simulink model "P4Model"  (R2023b)
settings: Solver=FixedStepAuto  StartTime=0.0  StopTime=3600  FixedStep=0.1  RelTol=1e-3
values from neighbouring files (symbols this model uses):
  psi = [0]    [Project2Init.m]
  x = [0]    [Project2Init.m]
  y = [0]    [Project2Init.m]
undefined symbols (not defined in the file or in its folder): batData, carData, motorData, rps2rpm
libraries: slpidlib x1
settings Model: Creator=ronal  LastModifiedBy=ronal
settings DebuggingCC: AlgebraicLoopMsg=none

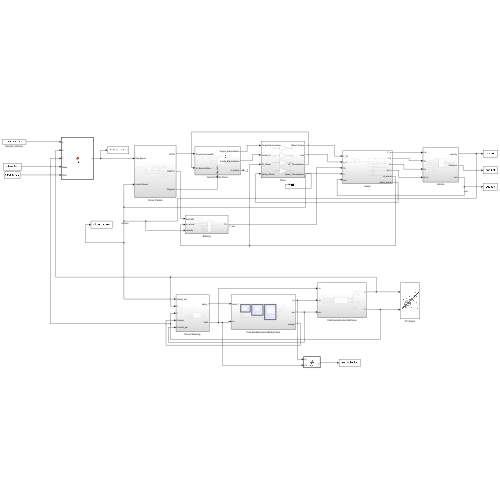
[thumbnail: Simulink's stored preview of the top-level diagram]
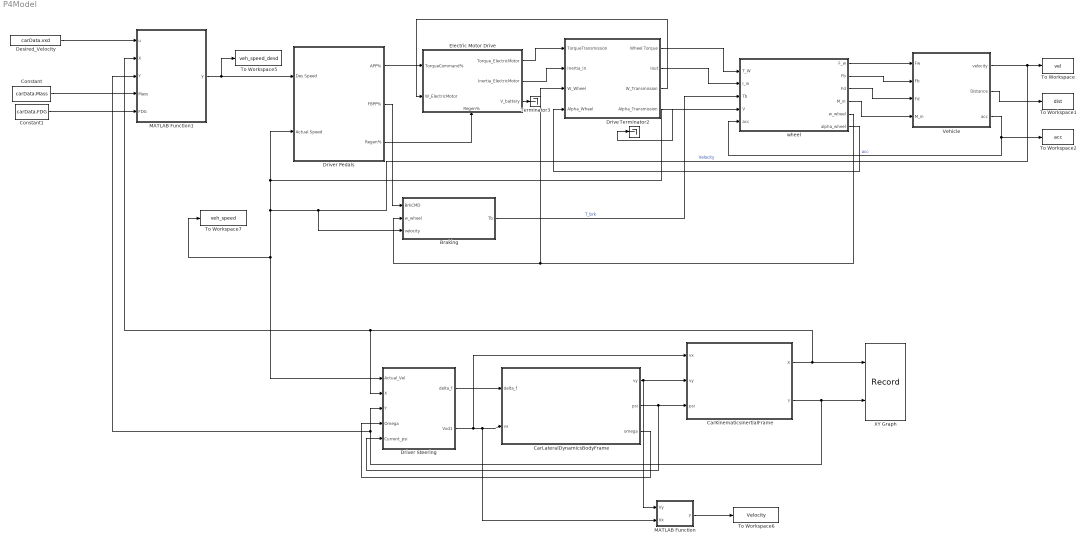
== system P4Model ==
  Braking : Subsystem
  CarKinematicsInertialFrame : Subsystem
  CarLateralDynamicsBodyFrame : Subsystem
  Constant : Constant  Value=carData.Mass
  Constant1 : Constant  Value=carData.FDG
  Desired_Velocity : Constant  Value=carData.vxd
  Drive : Subsystem
  "Driver Pedals " : Subsystem
  Driver Steering : Subsystem
  Electric Motor Drive : Subsystem
      settings: PortSchema="{\"entries\":[{\"content\":{\"sides\":[{\"content\":{\"connectorIds\":[\"In1\",\"In2\"]},\"type\":\"ConnectorPlacement.EquallySpacedRectSide\",\"uuid\":\"06f5b496-3bf6-4a8b-aebb-c7eaab5f1ccf\"},{\"content\":{\"connectorIds\":[\"Out1\",\"Out2\",\"Out3\"],\"side\":\"RIGHT\"},\"type\":\"ConnectorPlacement.EquallySpacedRectSide\",\"uuid\":\"1c240108-0efa-470d-9e35-d17d0925c84e\"},{\"content\":{\"side\":\"TOP\"},\"type\":\"ConnectorPlacement.EquallySpacedRectSide\",\"uuid\":\"0076995f-d270-4ea1-a86d-c1644fbb58c6\"},{\"content\":{\"connectorIds\":[\"In3\"],\"side\":\"BOTTOM\"},\"type\":\"ConnectorPlacement.EquallySpacedRectSide\",\"uuid\":\"f7a02404-3e3b-4c45-bbfb-e79306aab2e1\"}]},\"type\":\"ConnectorPlacement.EquallySpacedConnector\",\"uuid\":\"8c37f1ab-19c5-40e9-996c-a411e99a53bc\"}],\"packageUris\":[\"http://schema.mathworks.com/mf0/Connector/R2020b\"],\"version\":\"1.0\"}"
  MATLAB Function : MATLAB Function  TreatAsAtomicUnit=on
  MATLAB Function1 : MATLAB Function  TreatAsAtomicUnit=on
  Terminator2 : Terminator
  Terminator3 : Terminator
  To Workspace : ToWorkspace  VariableName=vel  SaveFormat=Timeseries  SampleTime=-1
  To Workspace1 : ToWorkspace  VariableName=dist  SaveFormat=Timeseries  SampleTime=-1
  To Workspace2 : ToWorkspace  VariableName=acc  SaveFormat=Timeseries  SampleTime=-1
  To Workspace5 : ToWorkspace  VariableName=veh_speed_desd  SaveFormat=Timeseries  SampleTime=-1
  To Workspace6 : ToWorkspace  VariableName=Velocity  SaveFormat=Timeseries  SampleTime=-1
  To Workspace7 : ToWorkspace  VariableName=veh_speed  SaveFormat=Timeseries  SampleTime=-1
  Vehicle : Subsystem
  XY Graph : Record  FileSettingsInternal="{\"entries\":[{\"content\":{\"excelSettings\":{\"content\":{},\"type\":\"Streamout.ExcelSettings\"}},\"type\":\"Streamout.FileSettingStorage\",\"uuid\":\"\"}],\"packageUris\":[\"http:\\/\\/schema.mathworks.com\\/mf0\\/streamout_blocks\\/R2020a\"],\"version\":\"1.0\"}"  Layout=[1 1]  SignalsInternal="{\"entries\":[{\"content\":{\"signals\":[{\"content\":{\"blockPath\":[],\"dimensions\":[1],\"domain\":\"\",\"lineColor\":\"#0072bd\",\"plots\":[1],\"port\":1,\"sid\":[\"\"],\"signalID\":2554,\"signalName\":\"CarKinematicsInertialFrame:1\"},\"type\":\"RecordBlkView.Signal\",\"uuid\":\"\"},{\"content\":{\"blockPath\":[],\"dimensions\":[1],\"domain\":\"\",\"lineColor\":\"#ff13a6\",\"plots\":[1],\"port\":2,\"sid\":[\"\"],\"signalID\":2558,\"signalName\":\"CarKinematicsInertialFrame:2\"},\"type\":\"RecordBlkView.Signal\",\"uuid\":\"\"}]},\"type\":\"RecordBlkView.InputSignals\",\"uuid\":\"\"}],\"packageUris\":[\"http:\\/\\/schema.mathworks.com\\/mf0\\/streamout_blocks\\/R2020a\"],\"version\":\"1.0\"}"  VisualizationBindings="{\"xyplotplugin\":{\"info\":[{\"series\":[{\"bindingParametersList\":[{\"parameter\":\"Y-Axis\",\"signalID\":2558,\"signalName\":\"CarKinematicsInertialFrame:2\"},{\"parameter\":\"X-Axis\",\"signalID\":2554,\"signalName\":\"CarKinematicsInertialFrame:1\"}],\"seriesID\":48790}],\"subplotID\":1}]}}"  CompatibilityTag=XY  st=-1
  "wheel " : Subsystem
  wires:
  CarKinematicsInertialFrame/2(Y) -> MATLAB Function1/3(Y), Driver Steering/3(Y), XY Graph/2
  Driver Steering/1(delta_f) -> CarLateralDynamicsBodyFrame/1(delta_f)
  Vehicle/3(acc) -> "wheel "/5(acc), To Workspace2/1  "acc"
  CarLateralDynamicsBodyFrame/2(psi) -> Driver Steering/5(Current_psi), CarKinematicsInertialFrame/3(psi)
  Driver Steering/2(Vxd1) -> CarKinematicsInertialFrame/1(vx), CarLateralDynamicsBodyFrame/2(vx), MATLAB Function/2(Vx)
  Drive/2(Iout) -> "wheel "/2(I_in)
  MATLAB Function/1(y) -> To Workspace6/1
  Constant1/1 -> MATLAB Function1/5(FDG)
  MATLAB Function1/1(y) -> "Driver Pedals "/1("Des Speed "), To Workspace5/1
  "wheel "/1(F_w) -> Vehicle/1("Fw ")
  Desired_Velocity/1 -> MATLAB Function1/1(u)
  "Driver Pedals "/1(APP%) -> Electric Motor Drive/1(TorqueCommand%)
  Electric Motor Drive/2(Inertia_ElectricMotor) -> Drive/2(Inertia_In)
  CarKinematicsInertialFrame/1(X) -> XY Graph/1, Driver Steering/2(X), MATLAB Function1/2(X)
  "Driver Pedals "/2("FBPP% ") -> Braking/1("BrkCMD ")
  CarLateralDynamicsBodyFrame/3(omega) -> Driver Steering/4(Omega)
  Drive/3(W_Transmission) -> Electric Motor Drive/2(W_ElectricMotor)
  CarLateralDynamicsBodyFrame/1(vy) -> CarKinematicsInertialFrame/2(vy), MATLAB Function/1(Vy)
  Vehicle/2("Distance ") -> To Workspace1/1
  Constant/1 -> MATLAB Function1/4(Mass)
  Drive/4(Alpha_Transmission) -> Terminator2/1
  Drive/1(Wheel Torque) -> "wheel "/1(T_W)
  "wheel "/5(w_wheel) -> Braking/2(w_wheel), Drive/3(W_Wheel)
  "wheel "/3(Fd) -> Vehicle/3(Fd)
  "wheel "/4(M_in) -> Vehicle/4("M_in ")
  Braking/1("Tb ") -> "wheel "/3(Tb)  "T_brk"
  Electric Motor Drive/1(Torque_ElectricMotor) -> Drive/1(TorqueTransmission)
  "Driver Pedals "/3(Regen%) -> Electric Motor Drive/3(Regen%)
  Vehicle/1("velocity ") -> "wheel "/4(V), "Driver Pedals "/2(Actual Speed), To Workspace7/1, Driver Steering/1(Actual_Vel), Braking/3("velocity "), To Workspace/1  "Velocity"
  "wheel "/6(alpha_wheel) -> Drive/4(Alpha_Wheel)
  "wheel "/2("Fb ") -> Vehicle/2("Fb ")
  Electric Motor Drive/3(V_battery) -> Terminator3/1

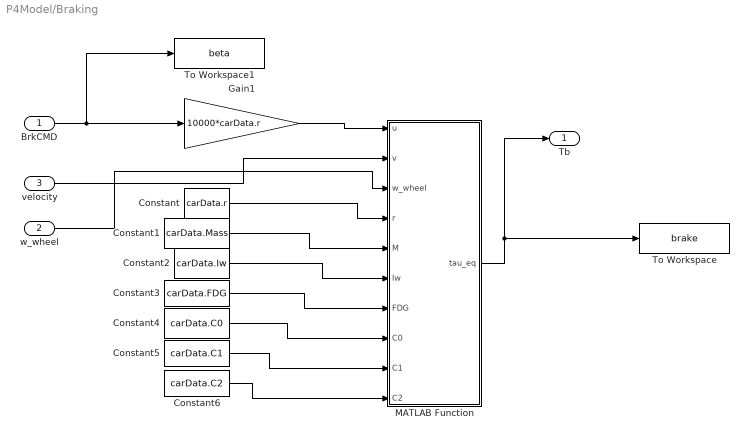
== system P4Model/Braking ==
  "BrkCMD " : Inport
  w_wheel : Inport  Port=2
  "velocity " : Inport  Port=3
  Constant : Constant  Value=carData.r
  Constant1 : Constant  Value=carData.Mass
  Constant2 : Constant  Value=carData.Iw
  Constant3 : Constant  Value=carData.FDG
  Constant4 : Constant  Value=carData.C0
  Constant5 : Constant  Value=carData.C1
  Constant6 : Constant  Value=carData.C2
  Gain1 : Gain  Gain=10000*carData.r
  MATLAB Function : MATLAB Function  TreatAsAtomicUnit=on
  To Workspace : ToWorkspace  VariableName=brake  SaveFormat=Timeseries  SampleTime=-1
  To Workspace1 : ToWorkspace  VariableName=beta  SaveFormat=Timeseries  SampleTime=-1
  "Tb " : Outport  VectorParamsAs1DForOutWhenUnconnected=off
  wires:
  "BrkCMD "/1 -> To Workspace1/1, Gain1/1
  Gain1/1 -> MATLAB Function/1(u)
  MATLAB Function/1(tau_eq) -> To Workspace/1, "Tb "/1
  "velocity "/1 -> MATLAB Function/2(v)
  Constant/1 -> MATLAB Function/4(r)
  Constant1/1 -> MATLAB Function/5(M)
  Constant2/1 -> MATLAB Function/6(Iw)
  Constant3/1 -> MATLAB Function/7(FDG)
  Constant4/1 -> MATLAB Function/8(C0)
  Constant5/1 -> MATLAB Function/9(C1)
  Constant6/1 -> MATLAB Function/10(C2)
  w_wheel/1 -> MATLAB Function/3(w_wheel)

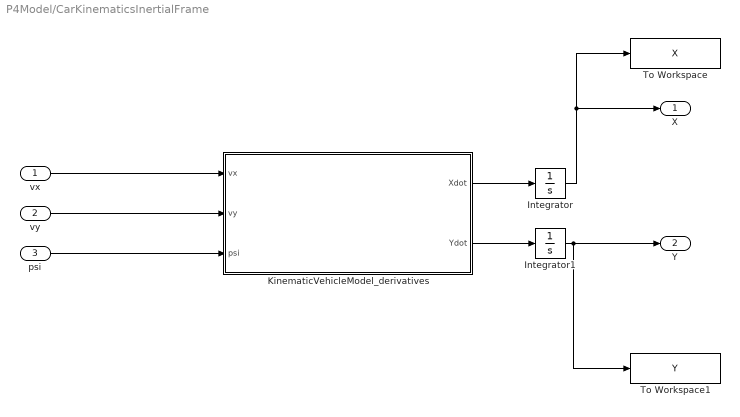
== system P4Model/CarKinematicsInertialFrame ==
  vx : Inport
  vy : Inport  Port=2
  psi : Inport  Port=3
  Integrator : Integrator  InitialCondition=carData.init.X0
  Integrator1 : Integrator  InitialCondition=carData.init.Y0
  KinematicVehicleModel_derivatives : MATLAB Function  TreatAsAtomicUnit=on  mask{obj=carData}
      mask prompts: obj "obj structure"
  To Workspace : ToWorkspace  VariableName=X  SaveFormat=Timeseries  SampleTime=-1
  To Workspace1 : ToWorkspace  VariableName=Y  SaveFormat=Timeseries  SampleTime=-1
  X : Outport
  Y : Outport  Port=2
  wires:
  KinematicVehicleModel_derivatives/1(Xdot) -> Integrator/1
  KinematicVehicleModel_derivatives/2(Ydot) -> Integrator1/1
  Integrator/1 -> To Workspace/1, X/1
  vx/1 -> KinematicVehicleModel_derivatives/1(vx)
  vy/1 -> KinematicVehicleModel_derivatives/2(vy)
  psi/1 -> KinematicVehicleModel_derivatives/3(psi)
  Integrator1/1 -> To Workspace1/1, Y/1

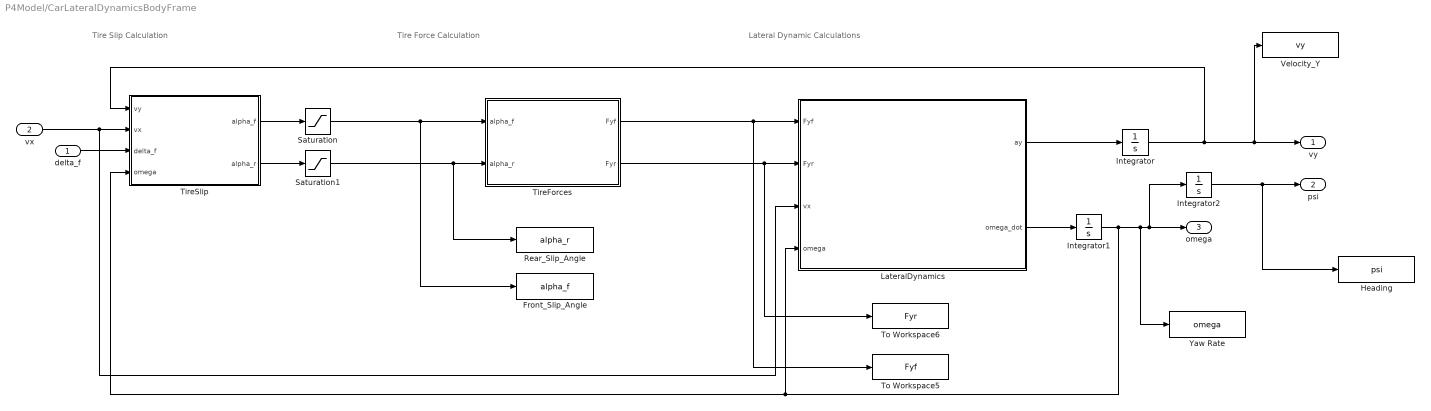
== system P4Model/CarLateralDynamicsBodyFrame ==
  note: Tire Slip Calculation
  note: Tire Force Calculation
  note: Lateral Dynamic Calculations
  delta_f : Inport
  vx : Inport  Port=2
  Front_Slip_Angle : ToWorkspace  VariableName=alpha_f  SaveFormat=Timeseries  SampleTime=-1
  Heading : ToWorkspace  VariableName=psi  SaveFormat=Timeseries  SampleTime=-1
  Integrator : Integrator  InitialCondition=carData.init.vy0
  Integrator1 : Integrator  InitialCondition=carData.init.omega0
  Integrator2 : Integrator  InitialCondition=carData.init.psi0
  LateralDynamics : MATLAB Function  TreatAsAtomicUnit=on  mask{obj=carData}
      mask prompts: obj "obj structure"
  Rear_Slip_Angle : ToWorkspace  VariableName=alpha_r  SaveFormat=Timeseries  SampleTime=-1
  Saturation : Saturate  UpperLimit=carData.maxAlpha  LowerLimit=-carData.maxAlpha
  Saturation1 : Saturate  UpperLimit=carData.maxAlpha  LowerLimit=-carData.maxAlpha
  TireForces : MATLAB Function  TreatAsAtomicUnit=on  mask{obj=carData}
      mask prompts: obj "obj structure"
  TireSlip : MATLAB Function  TreatAsAtomicUnit=on  mask{obj=carData}
      mask prompts: obj "obj structure"
  To Workspace5 : ToWorkspace  VariableName=Fyf  SaveFormat=Timeseries  SampleTime=-1
  To Workspace6 : ToWorkspace  VariableName=Fyr  SaveFormat=Timeseries  SampleTime=-1
  Velocity_Y : ToWorkspace  VariableName=vy  SaveFormat=Timeseries  SampleTime=-1
  Yaw Rate : ToWorkspace  VariableName=omega  SaveFormat=Timeseries  SampleTime=-1
  vy : Outport
  psi : Outport  Port=2
  omega : Outport  Port=3
  wires:
  LateralDynamics/1(ay) -> Integrator/1
  Integrator/1 -> vy/1, Velocity_Y/1, TireSlip/1(vy)
  LateralDynamics/2(omega_dot) -> Integrator1/1
  Integrator1/1 -> Integrator2/1, omega/1, Yaw Rate/1, LateralDynamics/4(omega), TireSlip/4(omega)
  TireSlip/1(alpha_f) -> Saturation/1
  TireSlip/2(alpha_r) -> Saturation1/1
  TireForces/1(Fyf) -> LateralDynamics/1(Fyf), To Workspace5/1
  TireForces/2(Fyr) -> LateralDynamics/2(Fyr), To Workspace6/1
  Saturation/1 -> TireForces/1(alpha_f), Front_Slip_Angle/1
  Saturation1/1 -> TireForces/2(alpha_r), Rear_Slip_Angle/1
  vx/1 -> TireSlip/2(vx), LateralDynamics/3(vx)
  delta_f/1 -> TireSlip/3(delta_f)
  Integrator2/1 -> Heading/1, psi/1

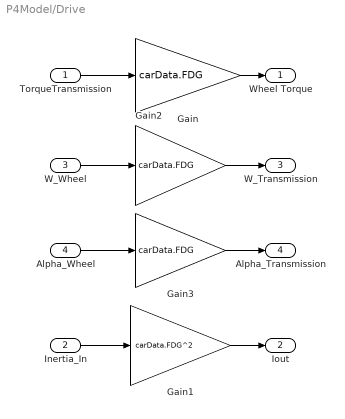
== system P4Model/Drive ==
  TorqueTransmission : Inport
  Inertia_In : Inport  Port=2
  W_Wheel : Inport  Port=3
  Alpha_Wheel : Inport  Port=4
  Gain : Gain  Gain=carData.FDG
  Gain1 : Gain  Gain=carData.FDG^2
  Gain2 : Gain  Gain=carData.FDG
  Gain3 : Gain  Gain=carData.FDG
  Wheel Torque : Outport
  Iout : Outport  Port=2
  W_Transmission : Outport  Port=3
  Alpha_Transmission : Outport  Port=4
  wires:
  TorqueTransmission/1 -> Gain/1
  Gain2/1 -> W_Transmission/1
  W_Wheel/1 -> Gain2/1
  Gain1/1 -> Iout/1
  Alpha_Wheel/1 -> Gain3/1
  Inertia_In/1 -> Gain1/1
  Gain3/1 -> Alpha_Transmission/1
  Gain/1 -> Wheel Torque/1

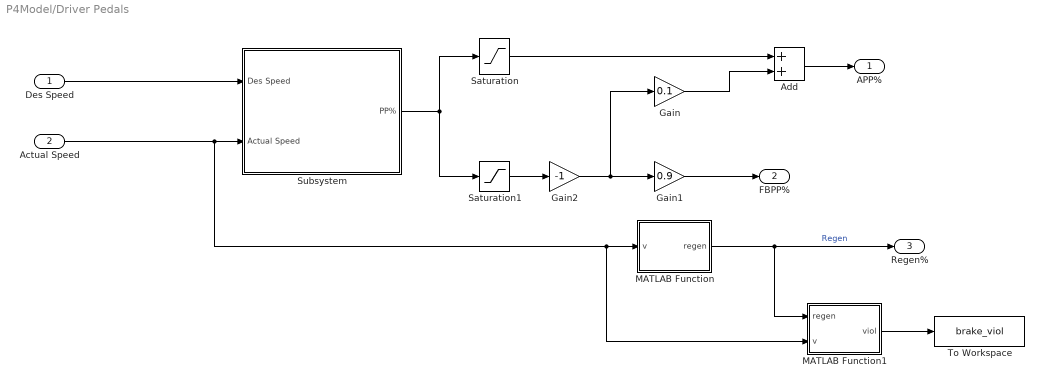
== system P4Model/Driver Pedals  ==
  "Des Speed " : Inport
  Actual Speed : Inport  Port=2
  Add : Sum
  Gain : Gain  Gain=0.1
  Gain1 : Gain  Gain=0.9
  Gain2 : Gain  Gain=-1
  MATLAB Function : MATLAB Function  TreatAsAtomicUnit=on
  MATLAB Function1 : MATLAB Function  TreatAsAtomicUnit=on
  Saturation : Saturate  UpperLimit=100  LowerLimit=0
  Saturation1 : Saturate  UpperLimit=0  LowerLimit=-100
  Subsystem : Subsystem
  To Workspace : ToWorkspace  VariableName=brake_viol  SaveFormat=Timeseries  SampleTime=-1
  APP% : Outport
  "FBPP% " : Outport  Port=2
  Regen% : Outport  Port=3
  wires:
  "Des Speed "/1 -> Subsystem/1("Des Speed ")
  Actual Speed/1 -> MATLAB Function1/2(v), MATLAB Function/1(v), Subsystem/2(Actual Speed)
  Subsystem/1(PP%) -> Saturation1/1, Saturation/1
  Add/1 -> APP%/1
  Saturation/1 -> Add/1
  Saturation1/1 -> Gain2/1
  Gain2/1 -> Gain/1, Gain1/1
  Gain1/1 -> "FBPP% "/1
  Gain/1 -> Add/2
  MATLAB Function/1(regen) -> MATLAB Function1/1(regen), Regen%/1  "Regen"
  MATLAB Function1/1(viol) -> To Workspace/1

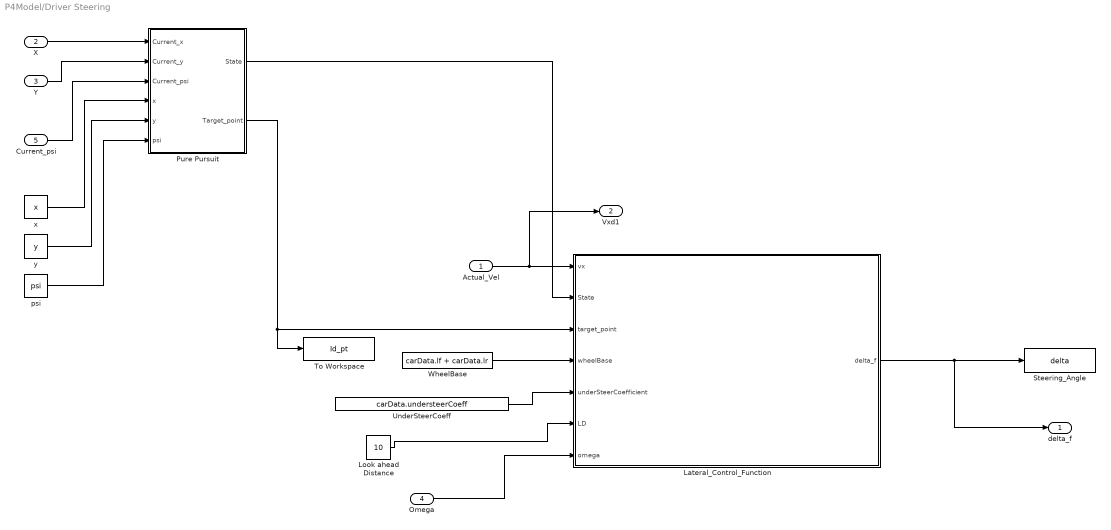
== system P4Model/Driver Steering ==
  Actual_Vel : Inport
  X : Inport  Port=2
  Y : Inport  Port=3
  Omega : Inport  Port=4
  Current_psi : Inport  Port=5
  Lateral_Control_Function : MATLAB Function  TreatAsAtomicUnit=on
  Look ahead Distance : Constant  Value=10
  Pure Pursuit : MATLAB Function  TreatAsAtomicUnit=on
  Steering_Angle : ToWorkspace  VariableName=delta  SaveFormat=Timeseries  SampleTime=-1
  To Workspace : ToWorkspace  VariableName=Id_pt  SaveFormat=Timeseries  SampleTime=-1
  UnderSteerCoeff : Constant  Value=carData.understeerCoeff
  WheelBase : Constant  Value=carData.lf + carData.lr
  psi : Constant  Value=psi
  x : Constant  Value=x
  y : Constant  Value=y
  delta_f : Outport
  Vxd1 : Outport  Port=2
  wires:
  Actual_Vel/1 -> Lateral_Control_Function/1(vx), Vxd1/1
  WheelBase/1 -> Lateral_Control_Function/4(wheelBase)
  UnderSteerCoeff/1 -> Lateral_Control_Function/5(underSteerCoefficient)
  Look ahead Distance/1 -> Lateral_Control_Function/6(LD)
  Omega/1 -> Lateral_Control_Function/7(omega)
  X/1 -> Pure Pursuit/1(Current_x)
  Y/1 -> Pure Pursuit/2(Current_y)
  Pure Pursuit/1(State) -> Lateral_Control_Function/2(State)
  Pure Pursuit/2(Target_point) -> To Workspace/1, Lateral_Control_Function/3(target_point)
  x/1 -> Pure Pursuit/4(x)
  y/1 -> Pure Pursuit/5(y)
  psi/1 -> Pure Pursuit/6(psi)
  Current_psi/1 -> Pure Pursuit/3(Current_psi)
  Lateral_Control_Function/1(delta_f) -> Steering_Angle/1, delta_f/1

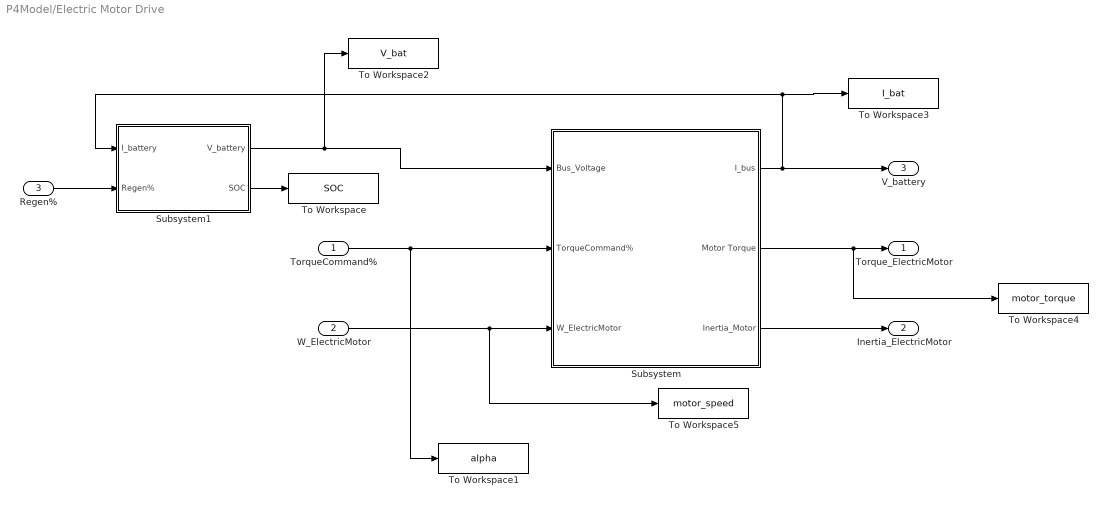
== system P4Model/Electric Motor Drive ==
  TorqueCommand% : Inport
  W_ElectricMotor : Inport  Port=2
  Regen% : Inport  Port=3
  Subsystem : Subsystem
  Subsystem1 : Subsystem
  To Workspace : ToWorkspace  VariableName=SOC  SaveFormat=Timeseries  SampleTime=-1
  To Workspace1 : ToWorkspace  VariableName=alpha  SaveFormat=Timeseries  SampleTime=-1
  To Workspace2 : ToWorkspace  VariableName=V_bat  SaveFormat=Timeseries  SampleTime=-1
  To Workspace3 : ToWorkspace  VariableName=I_bat  SaveFormat=Timeseries  SampleTime=-1
  To Workspace4 : ToWorkspace  VariableName=motor_torque  SaveFormat=Timeseries  SampleTime=-1
  To Workspace5 : ToWorkspace  VariableName=motor_speed  SaveFormat=Timeseries  SampleTime=-1
  Torque_ElectricMotor : Outport
  Inertia_ElectricMotor : Outport  Port=2
  V_battery : Outport  Port=3
  wires:
  TorqueCommand%/1 -> To Workspace1/1, Subsystem/2(TorqueCommand%)
  W_ElectricMotor/1 -> To Workspace5/1, Subsystem/3(W_ElectricMotor)
  Subsystem/2(Motor Torque) -> To Workspace4/1, Torque_ElectricMotor/1
  Subsystem/3(Inertia_Motor) -> Inertia_ElectricMotor/1
  Subsystem/1(I_bus) -> V_battery/1, To Workspace3/1, Subsystem1/1(I_battery)
  Subsystem1/1(V_battery) -> Subsystem/1(Bus_Voltage), To Workspace2/1
  Subsystem1/2(SOC) -> To Workspace/1
  Regen%/1 -> Subsystem1/2(Regen%)

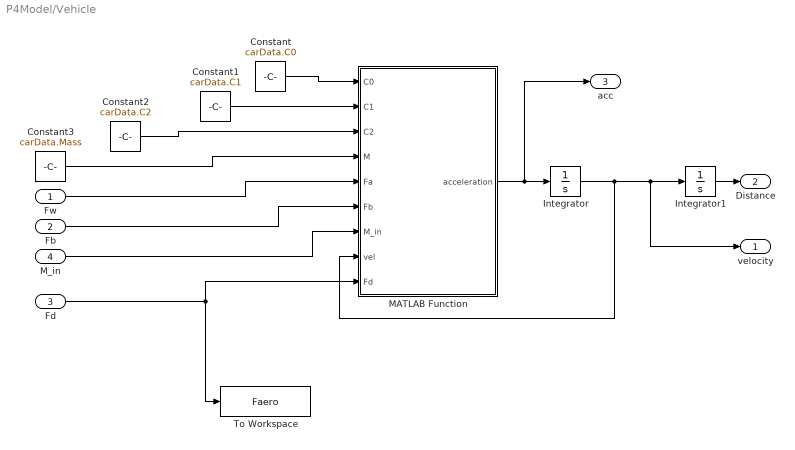
== system P4Model/Vehicle ==
  "Fw " : Inport
  "Fb " : Inport  Port=2
  Fd : Inport  Port=3
  "M_in " : Inport  Port=4
  Constant : Constant  Value=carData.C0
  Constant1 : Constant  Value=carData.C1
  Constant2 : Constant  Value=carData.C2
  Constant3 : Constant  Value=carData.Mass
  Integrator : Integrator  LimitOutput=on  LowerSaturationLimit=0
  Integrator1 : Integrator
  MATLAB Function : MATLAB Function  TreatAsAtomicUnit=on
  To Workspace : ToWorkspace  VariableName=Faero  SaveFormat=Timeseries  SampleTime=-1
  "velocity " : Outport  VectorParamsAs1DForOutWhenUnconnected=off
  "Distance " : Outport  Port=2  VectorParamsAs1DForOutWhenUnconnected=off
  acc : Outport  Port=3
  wires:
  Constant1/1 -> MATLAB Function/2(C1)
  Constant/1 -> MATLAB Function/1(C0)
  MATLAB Function/1(acceleration) -> Integrator/1, acc/1
  Constant2/1 -> MATLAB Function/3(C2)
  Constant3/1 -> MATLAB Function/4(M)
  "Fw "/1 -> MATLAB Function/5(Fa)
  "Fb "/1 -> MATLAB Function/6(Fb)
  Integrator/1 -> MATLAB Function/8(vel), "velocity "/1, Integrator1/1
  Integrator1/1 -> "Distance "/1
  "M_in "/1 -> MATLAB Function/7(M_in)
  Fd/1 -> To Workspace/1, MATLAB Function/9(Fd)

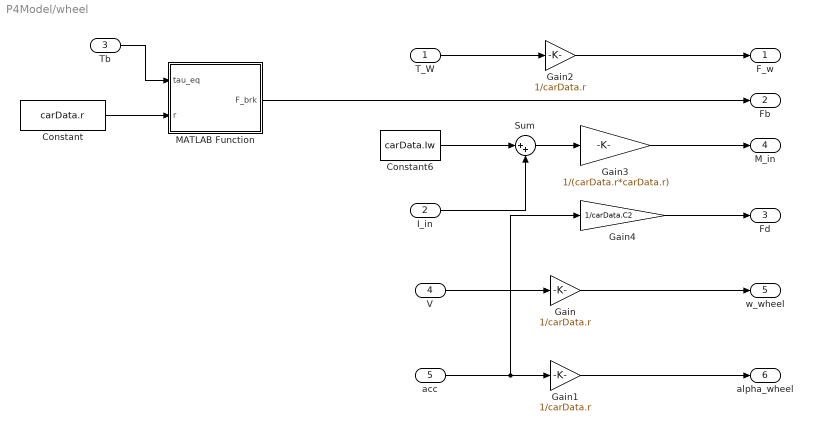
== system P4Model/wheel  ==
  T_W : Inport
  I_in : Inport  Port=2
  Tb : Inport  Port=3
  V : Inport  Port=4
  acc : Inport  Port=5
  Constant : Constant  Value=carData.r
  Constant6 : Constant  Value=carData.Iw
  Gain : Gain  Gain=1/carData.r
  Gain1 : Gain  Gain=1/carData.r
  Gain2 : Gain  Gain=1/carData.r
  Gain3 : Gain  Gain=1/(carData.r*carData.r)
  Gain4 : Gain  Gain=1/carData.C2
  MATLAB Function : MATLAB Function  TreatAsAtomicUnit=on
  Sum : Sum  Inputs=|++
  F_w : Outport
  "Fb " : Outport  Port=2
  Fd : Outport  Port=3
  M_in : Outport  Port=4
  w_wheel : Outport  Port=5
  alpha_wheel : Outport  Port=6
  wires:
  Gain/1 -> w_wheel/1
  V/1 -> Gain/1
  acc/1 -> Gain4/1, Gain1/1
  Gain1/1 -> alpha_wheel/1
  T_W/1 -> Gain2/1
  Gain2/1 -> F_w/1
  Gain3/1 -> M_in/1
  Constant6/1 -> Sum/1
  I_in/1 -> Sum/2
  Sum/1 -> Gain3/1
  MATLAB Function/1(F_brk) -> "Fb "/1
  Tb/1 -> MATLAB Function/1(tau_eq)
  Constant/1 -> MATLAB Function/2(r)
  Gain4/1 -> Fd/1

== system P4Model/Driver Pedals /Subsystem ==
  "Des Speed " : Inport
  Actual Speed : Inport  Port=2
  PID Controller : slpidlib/PID Controller  Controller=PID  Form=Parallel  TimeDomain=Continuous-time  UseExternalTs=off  SampleTime=-1  IntegratorMethod=Forward Euler  FilterMethod=Forward Euler  ControllerParametersSource=internal  P=0.1  I=0  UseKiTs=off  D=0  N=100  UseFilter=on  TunerSelectOption=Transfer Function Based (PID Tuner App)  InitialConditionSource=internal  InitialConditionForIntegrator=0  InitialConditionForFilter=0  DifferentiatorICPrevScaledInput=0  ExternalReset=none  TrackingMode=off  Kt=1  LimitOutput=on  SatLimitsSource=internal  UpperSaturationLimit=1  LowerSaturationLimit=-1  LinearizeAsGain=off  AntiWindupMode=none  Kb=1  LimitIntegrator=off  UpperIntegratorSaturationLimit=inf  LowerIntegratorSaturationLimit=-inf  POutMin=[]  POutMax=[]  IOutMin=[]  IOutMax=[]  DOutMin=[]  DOutMax=[]  NOutMin=[]  NOutMax=[]  SumOutMin=[]  SumOutMax=[]  SaturationOutMin=[]  SaturationOutMax=[]  PParamMin=[]  PParamMax=[]  IParamMin=[]  IParamMax=[]  DParamMin=[]  DParamMax=[]  NParamMin=[]  NParamMax=[]  KbParamMin=[]  KbParamMax=[]  KtParamMin=[]  KtParamMax=[]  KbOutMin=[]  KbOutMax=[]  KtOutMin=[]  KtOutMax=[]  IntegratorOutMin=[]  IntegratorOutMax=[]  FilterOutMin=[]  FilterOutMax=[]  SumI1OutMin=[]  SumI1OutMax=[]  SumI2OutMin=[]  SumI2OutMax=[]  SumI3OutMin=[]  SumI3OutMax=[]  SumI4OutMin=[]  SumI4OutMax=[]  SumDOutMin=[]  SumDOutMax=[]  DifferentiatorOutMin=[]  DifferentiatorOutMax=[]  FilterDiffOutCoefMin=[]  FilterDiffOutCoefMax=[]  ReciprocalOutMin=[]  ReciprocalOutMax=[]  SumDenOutMin=[]  SumDenOutMax=[]  SumNumOutMin=[]  SumNumOutMax=[]  DivideOutMin=[]  DivideOutMax=[]  UdiffTsProdOutMin=[]  UdiffTsProdOutMax=[]  NTsProdOutMin=[]  NTsProdOutMax=[]  UintegralTsProdOutMin=[]  UintegralTsProdOutMax=[]  UngainTsProdOutMin=[]  UngainTsProdOutMax=[]  ClampingZeroOutDataTypeStr=Inherit: Inherit via back propagation  ClampingZeroOutMin=[]  ClampingZeroOutMax=[]  FilterDenConstantOutDataTypeStr=Inherit: Inherit via back propagation  FilterDenConstantOutMin=[]  FilterDenConstantOutMax=[]  PCopyOutDataTypeStr=Inherit: Inherit via back propagation  PCopyOutMin=[]  PCopyOutMax=[]  NCopyOutDataTypeStr=Inherit: Inherit via back propagation  NCopyOutMin=[]  NCopyOutMax=[]  IntegratorContinuousStateAttributes=''  IntegratorStateMustResolveToSignalObject=off  IntegratorRTWStateStorageClass=Auto  FilterContinuousStateAttributes=''  FilterStateMustResolveToSignalObject=off  FilterRTWStateStorageClass=Auto  ParallelPVariant=InternalParameters  IdealPVariant=Disabled  IVariant=InternalParameters  DVariant=InternalParameters  IntegratorVariant=Continuous  SatVariant=Enabled  AWVariant=Passthrough  PCopyVariant=Disabled  TRVariant=Disabled  FdbkBlocksVariant=Forward  IdealPFdbkVariant=Disabled  SatFdbkVariant=Disabled  DerivativeFilterVariant=ContFilter  NVariant=InternalParameters  NCopyVariant=Disabled  FilterICVariant=InternalICsFilter  IntegratorICVariant=InternalICs  ExternalResetVariant=Disabled  TRSumVariant=Passthrough  SumFdbkVariant=Disabled  SumVariant=Sum_PID  TsampFilterVariant=InternalTs  TsampNgainVariant=Passthrough  TsampIntegralVariant=Disabled_SignalSpec  ExternalSaturationOutDataTypeStr=Inherit: Same as second input
  Sum : Sum  Inputs=|+-
  PP% : Outport
  wires:
  PID Controller/1 -> PP%/1
  Sum/1 -> PID Controller/1
  "Des Speed "/1 -> Sum/1
  Actual Speed/1 -> Sum/2

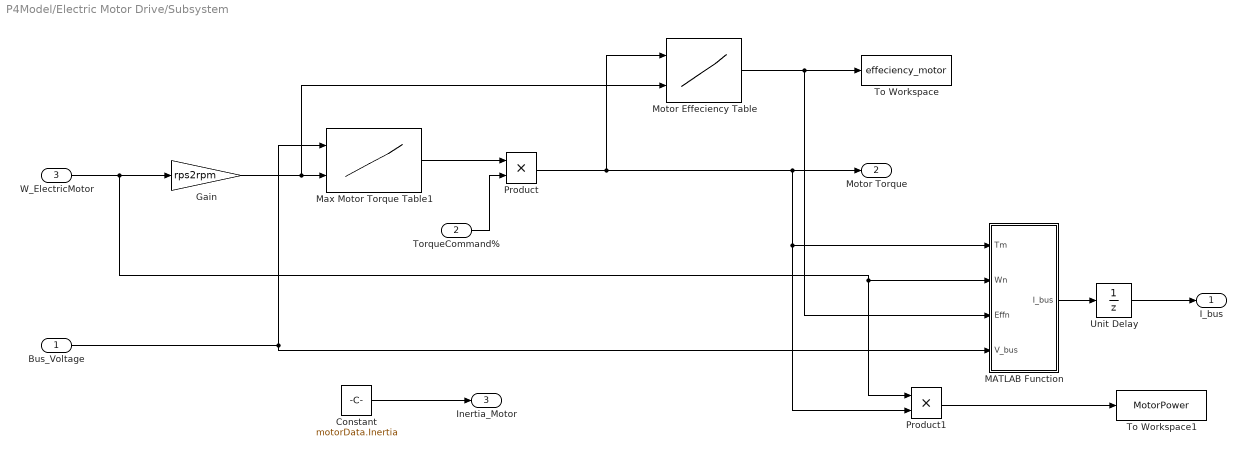
== system P4Model/Electric Motor Drive/Subsystem ==
  Bus_Voltage : Inport
  TorqueCommand% : Inport  Port=2
  W_ElectricMotor : Inport  Port=3
  Constant : Constant  Value=motorData.Inertia
  Gain : Gain  Gain=rps2rpm
  MATLAB Function : MATLAB Function  TreatAsAtomicUnit=on
  Max Motor Torque Table1 : Lookup_n-D  BreakpointsForDimension1=motorData.vbus  BreakpointsForDimension2=motorData.rpm  Table=motorData.maxtorque  InternalRulePriority=Speed  RndMeth=Simplest
      settings: InputPortMap=u0,u1
  Motor Effeciency Table : Lookup_n-D  BreakpointsForDimension1=motorData.eta_torque  BreakpointsForDimension2=motorData.eta_speed  Table=motorData.eta_val  InternalRulePriority=Speed  RndMeth=Simplest
      settings: InputPortMap=u0,u1
  Product : Product
  Product1 : Product
  To Workspace : ToWorkspace  VariableName=effeciency_motor  SaveFormat=Timeseries  SampleTime=-1
  To Workspace1 : ToWorkspace  VariableName=MotorPower  SaveFormat=Timeseries  SampleTime=-1
  Unit Delay : UnitDelay  SampleTime=-1  HasFrameUpgradeWarning=on
  I_bus : Outport
  Motor Torque : Outport  Port=2
  Inertia_Motor : Outport  Port=3
  wires:
  MATLAB Function/1(I_bus) -> Unit Delay/1
  Bus_Voltage/1 -> Max Motor Torque Table1/1, MATLAB Function/4(V_bus)
  W_ElectricMotor/1 -> Product1/1, MATLAB Function/2(Wn), Gain/1
  Gain/1 -> Motor Effeciency Table/2, Max Motor Torque Table1/2
  Max Motor Torque Table1/1 -> Product/1
  TorqueCommand%/1 -> Product/2
  Product/1 -> Product1/2, MATLAB Function/1(Tm), Motor Torque/1, Motor Effeciency Table/1
  Motor Effeciency Table/1 -> To Workspace/1, MATLAB Function/3(Effn)
  Product1/1 -> To Workspace1/1
  Constant/1 -> Inertia_Motor/1
  Unit Delay/1 -> I_bus/1

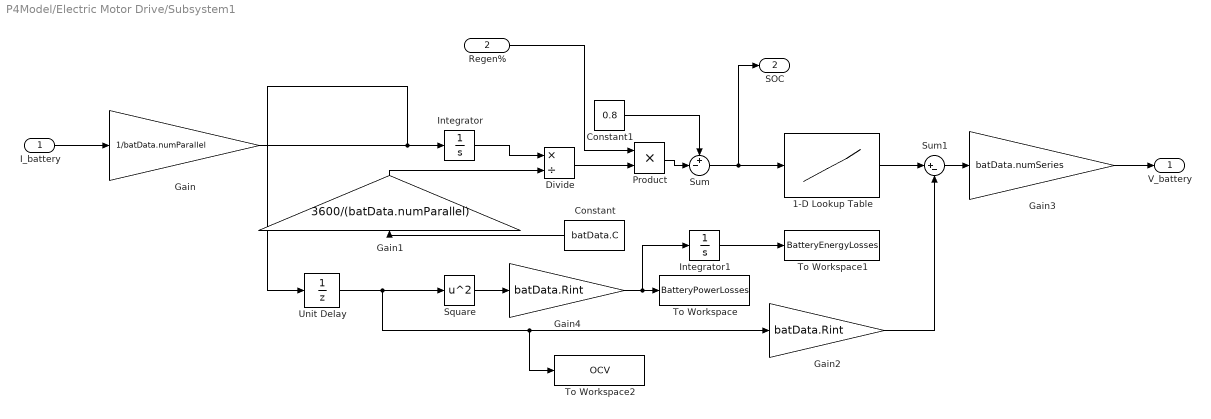
== system P4Model/Electric Motor Drive/Subsystem1 ==
  I_battery : Inport
  Regen% : Inport  Port=2
  1-D Lookup Table : Lookup_n-D  NumberOfTableDimensions=1  BreakpointsForDimension1=batData.SOC  Table=batData.OCV  InternalRulePriority=Speed  RndMeth=Simplest
  Constant : Constant  Value=batData.C
  Constant1 : Constant  Value=0.8
  Divide : Product  Inputs=*/
  Gain : Gain  Gain=1/batData.numParallel
  Gain1 : Gain  Gain=3600/(batData.numParallel)
  Gain2 : Gain  Gain=batData.Rint
  Gain3 : Gain  Gain=batData.numSeries
  Gain4 : Gain  Gain=batData.Rint
  Integrator : Integrator
  Integrator1 : Integrator
  Product : Product
  Square : Math  Operator=square
  Sum : Sum  Inputs=+-|
  Sum1 : Sum  Inputs=|+-
  To Workspace : ToWorkspace  VariableName=BatteryPowerLosses  SaveFormat=Timeseries  SampleTime=-1
  To Workspace1 : ToWorkspace  VariableName=BatteryEnergyLosses  SaveFormat=Timeseries  SampleTime=-1
  To Workspace2 : ToWorkspace  VariableName=OCV  SaveFormat=Timeseries  SampleTime=-1
  Unit Delay : UnitDelay  SampleTime=-1  HasFrameUpgradeWarning=on
  V_battery : Outport
  SOC : Outport  Port=2
  wires:
  I_battery/1 -> Gain/1
  Gain/1 -> Unit Delay/1, Integrator/1
  Gain1/1 -> Divide/2
  Sum1/1 -> Gain3/1
  Unit Delay/1 -> To Workspace2/1, Gain2/1, Square/1
  Constant/1 -> Gain1/1
  Square/1 -> Gain4/1
  Integrator/1 -> Divide/1
  Constant1/1 -> Sum/1
  Gain4/1 -> To Workspace/1, Integrator1/1
  Sum/1 -> SOC/1, 1-D Lookup Table/1
  Integrator1/1 -> To Workspace1/1
  1-D Lookup Table/1 -> Sum1/1
  Gain2/1 -> Sum1/2
  Gain3/1 -> V_battery/1
  Divide/1 -> Product/2
  Product/1 -> Sum/2
  Regen%/1 -> Product/1

== matlab function P4Model/CarLateralDynamicsBodyFrame/TireForces ==
  data: alpha_f input; alpha_r input; Fyf output; carData parameter; Fyr output
function [Fyf, Fyr] = fcn(alpha_f, alpha_r, carData)

Fyf = min(carData.Fyfmax,carData.Calpha_f * alpha_f);
Fyr = min(carData.Fyrmax, carData.Calpha_r * alpha_r);
end

== matlab function P4Model/CarLateralDynamicsBodyFrame/TireSlip ==
  data: vy input size=1; vx input; delta_f input size=1; omega input; alpha_f output; carData parameter; alpha_r output
function [alpha_f, alpha_r] = fcn(vy,  vx, delta_f, omega, carData) %omega is psi dot


if abs(vx)> carData.vx_threshold1
      alpha_f = delta_f - atan(vy + omega * carData.lf) / vx; %might need an arctan
      alpha_r = - atan(vy - omega * carData.lr) / vx; %might need an arctan
else
      alpha_f = 0;
      alpha_r = 0;
end



end

== matlab function P4Model/Driver Steering/Lateral_Control_Function ==
  data: vx input; State input; target_point input; wheelBase input; underSteerCoefficient input; LD input; omega input; delta_f output
function delta_f   = latControl(vx,State,target_point,wheelBase, underSteerCoefficient, LD, omega)

current_x = State(1);
current_y = State(2);
current_psi = State(3);

target_x = target_point(1);
target_y = target_point(2);
target_psi = target_point(3);

distances = vecnorm(target_point(:,1:2)'-State(1:2));
[~,min_index] = min(distances);

target_index = min_index;

for i = target_index:length(target_point)
    dist = norm(target_point(i,1:2)'-State(1:2)');
    
    if dist > LD
        break
    end
end


if target_index > length(target_x)
    target_index = length(target_x);
end

target_x = target_point(i,1);
target_y = target_point(i,2);

alpha = atan2(target_y-current_y,target_x-current_x) - current_psi;
psi_dot_d = (2*wheelBase*sin(alpha))/LD;
delta_f =(psi_dot_d-omega);

== matlab function P4Model/Driver Pedals /MATLAB Function ==
  data: regen output; v input
function regen = fcn(v)

    speed = (3600/1600)*v;
    
    if speed < 5
        regen = 0;
        
    elseif speed == 25
        regen = 0.95;
        

    elseif v > 25
        regen = 0.95;
        
    else
        regen = ((0.95/20)*speed) - 0.2375;
    end

== matlab function P4Model/MATLAB Function ==
  data: Vy input; y output; Vx input
function y = fcn(Vy, Vx)

y = sqrt(Vy^2 + Vx^2);

== matlab function P4Model/Driver Pedals /MATLAB Function1 ==
  data: regen input; viol output; v input
function viol = violfcn(regen, v)

    speed = (3600/1600)*v;
    
    if speed < 5
        regen_vio = 0;
        if regen == regen_vio
            viol = 0;
        else
            viol = 1;
        end

    elseif speed == 25
        regen_vio = 0.95;
        if regen == regen_vio
            viol = 0;
        else
            viol = 1;
        end

    elseif v > 25
        regen_vio = 0.95;
        if regen == regen_vio
            viol = 0;
        else
            viol = 1;
        end
    else
        regen_vio = ((0.95/20)*speed) - 0.2375;
        if regen == regen_vio
            viol = 0;
        else
            viol = 1;
        end
    end

== matlab function P4Model/MATLAB Function1 ==
  data: u input; y output; X input; Y input; Mass input; FDG input
function y = fcn(u, X, Y, Mass, FDG)

y=8; % Min Speed
max_speed = 10; % Max Speed


Brake_Force = Mass * 9.81 * FDG;
Max_deceleration = Brake_Force/Mass;
Brake_distance = (max_speed^2)/(2*Max_deceleration);

if X > 0 && X < 900 - Brake_distance && Y > -100 %Conditions for straightaway 1
    y = max_speed;
end

if X > 0 + Brake_distance && X < 900  && Y < -100 % Conditions for straightaway 2
    y = max_speed;
end

== matlab function P4Model/Driver Steering/Pure Pursuit ==
  data: Current_x input; State output; Current_y input; Current_psi input; Target_point output; x input; y input; psi input
function [State,Target_point]= fcn(Current_x, Current_y, Current_psi, x, y, psi)

State = [Current_x; Current_y; Current_psi];
Target_point = [x,y,psi];

== matlab function P4Model/Vehicle/MATLAB Function ==
  data: C0 input; acceleration output; C1 input; C2 input; M input; Fa input; Fb input; M_in input; vel input; Fd input
function acceleration   = vehicle(C0,C1,C2,M,Fa,Fb,M_in, vel, Fd)

acceleration = (((Fa-(Fb+Fd)))-(C0+ C1*vel + C2*(vel)^2))/(M+M_in);

== matlab function P4Model/wheel /MATLAB Function ==
  data: tau_eq input; F_brk output; r input
function F_brk = fcn(tau_eq,r)


F_brk = tau_eq / r; % Braking force at the wheel
end

== matlab function P4Model/Electric Motor Drive/Subsystem/MATLAB Function ==
  data: Tm input; I_bus output; Wn input; Effn input; V_bus input
function I_bus = fcn(Tm,Wn,Effn,V_bus)

Pm = Tm*Wn;
sgn_m = Pm/(abs(Pm)+0.001);
Pe = Pm * (Effn^sgn_m);

if V_bus > 0
    I_bus = Pe/V_bus;
else
    I_bus = 0;
end

== matlab function P4Model/CarKinematicsInertialFrame/KinematicVehicleModel_derivatives ==
  data: vx input; vy input; psi input size=1; Xdot output; Ydot output
%{
Function "fcn" multiplies the body fixed frame
velocities vx and vy by the rotation matrix to get
global frame velocities Xdot and Ydot.

Function "TF" applies the rotation matrix 
taking yaw angle "psi" as input
%}
function [Xdot, Ydot] = fcn(vx, vy, psi)
    temp = TF(psi) * [vx;vy]; 
    Xdot = temp(1);
    Ydot = temp(2);
  
end

function y = TF(psi)
    y = [cos(psi), -sin(psi); sin(psi), cos(psi)];
end

== matlab function P4Model/CarLateralDynamicsBodyFrame/LateralDynamics ==
  data: Fyf input; Fyr input size=1; vx input; omega input; ay output; carData parameter; omega_dot output
function [ay, omega_dot] = fcn(Fyf, Fyr, vx, omega, carData) %omega is psi dot 

Fy = Fyf + Fyr;
ay = Fy / carData.Mass - omega * vx;
        
M  = Fyf * carData.lf - Fyr * carData.lr;        
omega_dot = M / carData.Inertia;        

end

== matlab function P4Model/Braking/MATLAB Function ==
  data: u input; tau_eq output; v input; w_wheel input; r input; M input; Iw input; FDG input; C0 input; C1 input; C2 input
%function y = fcn(u,v)
%y =u*sign(v)
%y = u * v/(abs(v)+0.001);
%y = u;

% Most values come from conditions in init script
% mu_b, alpha_b, g_b can be tuned to desired braking behavior

function tau_eq = fcn(u, v, w_wheel, r,M,Iw,FDG,C0,C1,C2)

% from init
%r = 0.36;
%M = 1000;
%Iw = 0.5*7*(r^2);
%FDG = 2.5;
%C0 = 0.0041;
%C1 = 0.000066;



% Effective Inertia (downstream perspective)
I_eq = Iw + (M / (w_wheel / v)^2); % Effective inertia from the downstream perspective

% Braking Torque Calculation
N_b_max = M * 9.81 * FDG; % Maximum brake normal force
alpha_b = u / 10000; % Brake command percentage (assuming the gain block scales the input from 0-1 to 0-10000)
mu_b = 0.7; % Friction coefficient (standard, can be tuned to whatever)
g_b = 0.5; % Geometric design factor (assuming a typical disk brake design)

if alpha_b == 0
    tau_b = 0; % No braking torque when brake command is zero
else
    N_b = alpha_b * N_b_max; % Actual brake normal force
    tau_b = mu_b * N_b * g_b * r; % Brake torque
end

% Braking Force Calculation
if v > 0 
    tau_eq = tau_b - (C0 + C1 * v + C2 * v^2) * (1 / (w_wheel / v)); % Effective downstream torque
else
    tau_eq = tau_b;
end
